simulink library "InterModuleProtocol"  (R2023b)
settings: Solver=VariableStepAuto  StartTime=0.0  StopTime=10.0  RelTol=1e-3
undefined symbols (not defined in the file or in its folder): accelerationNED, accelerationNEDXYZ, accelerationXYZ, angleOfAttack, courseOverGround, orientationQuaternion, orientationRollPitchYaw, positionLLA, positionNED, sideSlipAngle, speedOverGround, velocityNED, velocityNEDUVW, velocityPQR, velocityUVW
libraries: $bdroot x10
(part 2 of 3)

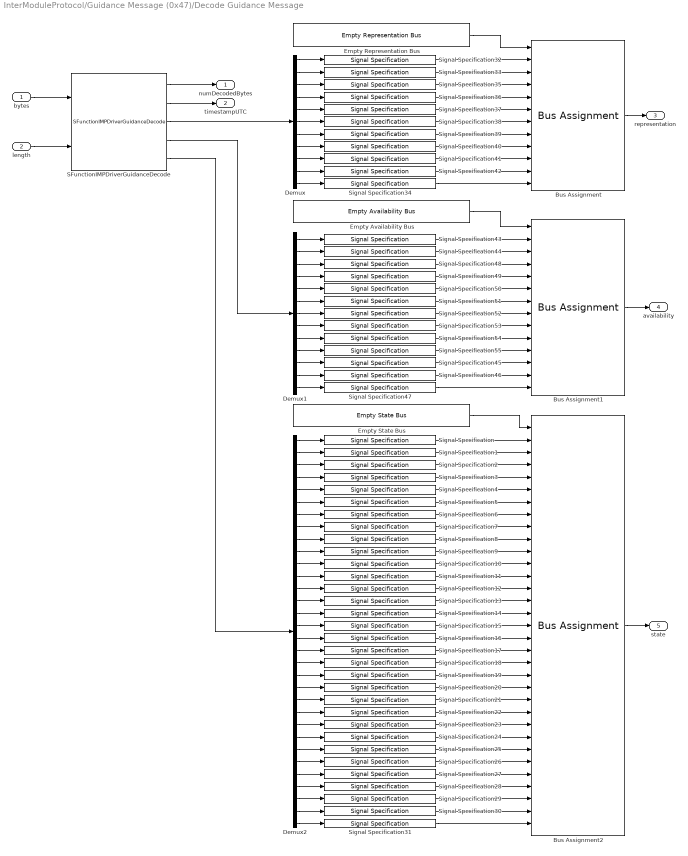
== system InterModuleProtocol/Guidance Message (0x47)/Decode Guidance Message ==
  bytes : Inport  OutDataTypeStr=uint8
  length : Inport  Port=2  OutDataTypeStr=uint32  PortDimensions=1
  Bus Assignment : BusAssignment  AssignedSignals=positionLLA,positionNED,orientationQuaternion,orientationRollPitchYaw,velocityNEDUVW,velocityPQR,accelerationNEDXYZ,courseOverGround,speedOverGround,angleOfAttack,sideSlipAngle
  Bus Assignment1 : BusAssignment  AssignedSignals=positionLLA,positionNED,orientationQuaternion,orientationRollPitchYaw,velocityNED,velocityUVW,velocityPQR,accelerationNED,accelerationXYZ,courseOverGround,speedOverGround,angleOfAttack,sideSlipAngle
  Bus Assignment2 : BusAssignment  AssignedSignals=positionLatitude,positionLongitude,positionAltitude,positionNorth,positionEast,positionDown,orientationQuaternionW,orientationQuaternionX,orientationQuaternionY,orientationQuaternionZ,orientationRoll,orientationPitch,orientationYaw,velocityNorth,velocityEast,velocityDown,velocityU,velocityV,velocityW,velocityP,velocityQ,velocityR,accelerationNorth,accelerationEast,accelerationDown,accelerationX,accelerationY,accelerationZ,courseOverGround,speedOverGround,angleOfAttack,sideSlipAngle
  Demux : Demux  Outputs=11
  Demux1 : Demux  Outputs=13
  Demux2 : Demux  Outputs=32
  Empty Availability Bus : $bdroot/Empty Availability Bus
  Empty Representation Bus : $bdroot/Empty Representation Bus
  Empty State Bus : $bdroot/Empty State Bus
  SFunctionIMPDriverGuidanceDecode : S-Function  FunctionName=SFunctionIMPDriverGuidanceDecode  Parameters=SampleTime  SFunctionDeploymentMode=off  EnableBusSupport=off  mask(Legacy Function){SFunctionSpec=void IMP_OutputDriverGuidanceDecode(uint8 u1[], uint32 u2, int32 y1[1], double y2[1], uint8 y3[11], uint8 y4[13], double y5[32]), SampleTime=-1, ShowSpec=off}
      mask prompts: SampleTime "Sample time (-1 for inherited):"; ShowSpec "Display function specification"
      mask help:
      | This block allows you to call the legacy functions specified by the following Legacy Code Tool definition:
      | def.SFunctionName = 'SFunctionIMPDriverGuidanceDecode';
      | def.OutputFcnSpec = 'void IMP_OutputDriverGuidanceDecode(uint8 u1[], uint32 u2, int32 y1[1], double y2[1], uint8 y3[11], uint8 y4[13], double y5[32])';
      | def.StartFcnSpec = 'void IMP_CreateDriverGuidanceDecode()';
      | def.TerminateFcnSpec = 'void IMP_DeleteDriverGuidanceDecode()';
      | def.HeaderFiles = {'IMP_DriverGuidanceDecode.h'};
      | def.SourceFiles = {'IMP_DriverGuidanceDecode.cpp', 'InterModuleProtocol.cpp', 'IMPConvexPolygon.cpp', 'IMPState.cpp', 'IMPStateConfiguration.cpp'};
      | def.IncPaths = {'..\..\source\InterModuleProtocol'};
      | def.SrcPaths = {'..\..\source\InterModuleProtocol'};
      | def.SampleTime = 'parameterized';
      | def.Options.useTlcWithAccel = false;
      mask Help: <p>This block was generated automatically by the Legacy Code Tool. For detailed help on this tool, call<a href="matlab:legacy_code('help')"> legacy_code('help')</a>.</p>
      mask Callback ShowSpec:
      | if strcmp(get_param(gcbh, 'ShowSpec'), 'on')
      |   set_param(gcbh, 'MaskDisplay', sprintf('fprintf(''%s'');', get_param(gcbh, 'SFunctionSpec')));
      | else
      |   set_param(gcbh, 'MaskDisplay', sprintf('fprintf(''%s'');', get_param(gcbh, 'FunctionName')));
      | end
      mask Display: fprintf('SFunctionIMPDriverGuidanceDecode');
  Signal Specification{,1,10..12,28,30..31} (8 alike) : SignalSpecification  OutDataTypeStr=double  Unit=rad  Dimensions=1
  Signal Specification{13..18,29} (7 alike) : SignalSpecification  OutDataTypeStr=double  Unit=m/s  Dimensions=1
  Signal Specification19 : SignalSpecification  OutDataTypeStr=double  Unit=rad/s  Dimensions=1
  Signal Specification{2..5} (4 alike) : SignalSpecification  OutDataTypeStr=double  Unit=m  Dimensions=1
  Signal Specification20 : SignalSpecification  OutDataTypeStr=double  Unit=rad/s  Dimensions=1
  Signal Specification21 : SignalSpecification  OutDataTypeStr=double  Unit=rad/s  Dimensions=1
  Signal Specification{22..27} (6 alike) : SignalSpecification  OutDataTypeStr=double  Unit=m/s^2  Dimensions=1
  Signal Specification{32..55} (24 alike) : SignalSpecification  OutDataTypeStr=uint8  Dimensions=1
  Signal Specification{6..9} (4 alike) : SignalSpecification  OutDataTypeStr=double  Dimensions=1
  numDecodedBytes : Outport  OutDataTypeStr=int32  PortDimensions=1  VectorParamsAs1DForOutWhenUnconnected=off
  timestampUTC : Outport  Port=2  OutDataTypeStr=double  Unit=s  PortDimensions=1  VectorParamsAs1DForOutWhenUnconnected=off
  representation : Outport  Port=3  VectorParamsAs1DForOutWhenUnconnected=off
  availability : Outport  Port=4  VectorParamsAs1DForOutWhenUnconnected=off
  state : Outport  Port=5  VectorParamsAs1DForOutWhenUnconnected=off
  wires:
  length/1 -> SFunctionIMPDriverGuidanceDecode/2
  SFunctionIMPDriverGuidanceDecode/2 -> timestampUTC/1
  bytes/1 -> SFunctionIMPDriverGuidanceDecode/1
  SFunctionIMPDriverGuidanceDecode/1 -> numDecodedBytes/1
  SFunctionIMPDriverGuidanceDecode/3 -> Demux/1
  SFunctionIMPDriverGuidanceDecode/4 -> Demux1/1
  Demux2/29 -> Signal Specification28/1
  Demux2/30 -> Signal Specification29/1
  Demux2/25 -> Signal Specification24/1
  Demux2/22 -> Signal Specification21/1
  Demux2/23 -> Signal Specification22/1
  Demux2/16 -> Signal Specification15/1
  Demux2/18 -> Signal Specification17/1
  Demux2/15 -> Signal Specification14/1
  Demux2/12 -> Signal Specification11/1
  Demux2/14 -> Signal Specification13/1
  Demux2/11 -> Signal Specification10/1
  Demux2/10 -> Signal Specification9/1
  Demux2/5 -> Signal Specification4/1
  Demux2/13 -> Signal Specification12/1
  Demux2/4 -> Signal Specification3/1
  Demux2/27 -> Signal Specification26/1
  Demux2/6 -> Signal Specification5/1
  Demux2/24 -> Signal Specification23/1
  Demux2/26 -> Signal Specification25/1
  Demux2/3 -> Signal Specification2/1
  Demux2/21 -> Signal Specification20/1
  Demux2/9 -> Signal Specification8/1
  Demux2/20 -> Signal Specification19/1
  Demux2/17 -> Signal Specification16/1
  Demux2/32 -> Signal Specification31/1
  Demux2/8 -> Signal Specification7/1
  Demux2/19 -> Signal Specification18/1
  Demux2/7 -> Signal Specification6/1
  Demux2/2 -> Signal Specification1/1
  Demux2/1 -> Signal Specification/1
  Demux2/28 -> Signal Specification27/1
  Demux2/31 -> Signal Specification30/1
  SFunctionIMPDriverGuidanceDecode/5 -> Demux2/1
  Empty Representation Bus/1 -> Bus Assignment/1
  Bus Assignment/1 -> representation/1
  Bus Assignment1/1 -> availability/1
  Empty Availability Bus/1 -> Bus Assignment1/1
  Empty State Bus/1 -> Bus Assignment2/1
  Signal Specification/1 -> Bus Assignment2/2
  Signal Specification1/1 -> Bus Assignment2/3
  Signal Specification2/1 -> Bus Assignment2/4
  Signal Specification3/1 -> Bus Assignment2/5
  Signal Specification4/1 -> Bus Assignment2/6
  Signal Specification5/1 -> Bus Assignment2/7
  Signal Specification6/1 -> Bus Assignment2/8
  Signal Specification7/1 -> Bus Assignment2/9
  Signal Specification8/1 -> Bus Assignment2/10
  Signal Specification9/1 -> Bus Assignment2/11
  Signal Specification10/1 -> Bus Assignment2/12
  Signal Specification11/1 -> Bus Assignment2/13
  Signal Specification12/1 -> Bus Assignment2/14
  Signal Specification13/1 -> Bus Assignment2/15
  Signal Specification14/1 -> Bus Assignment2/16
  Signal Specification15/1 -> Bus Assignment2/17
  Signal Specification16/1 -> Bus Assignment2/18
  Signal Specification17/1 -> Bus Assignment2/19
  Signal Specification18/1 -> Bus Assignment2/20
  Signal Specification19/1 -> Bus Assignment2/21
  Signal Specification20/1 -> Bus Assignment2/22
  Signal Specification21/1 -> Bus Assignment2/23
  Signal Specification22/1 -> Bus Assignment2/24
  Signal Specification23/1 -> Bus Assignment2/25
  Signal Specification24/1 -> Bus Assignment2/26
  Signal Specification25/1 -> Bus Assignment2/27
  Signal Specification26/1 -> Bus Assignment2/28
  Signal Specification27/1 -> Bus Assignment2/29
  Signal Specification28/1 -> Bus Assignment2/30
  Signal Specification29/1 -> Bus Assignment2/31
  Signal Specification30/1 -> Bus Assignment2/32
  Signal Specification31/1 -> Bus Assignment2/33
  Bus Assignment2/1 -> state/1
  Signal Specification32/1 -> Bus Assignment/2
  Signal Specification33/1 -> Bus Assignment/3
  Signal Specification35/1 -> Bus Assignment/4
  Signal Specification36/1 -> Bus Assignment/5
  Signal Specification37/1 -> Bus Assignment/6
  Signal Specification38/1 -> Bus Assignment/7
  Signal Specification39/1 -> Bus Assignment/8
  Signal Specification40/1 -> Bus Assignment/9
  Signal Specification41/1 -> Bus Assignment/10
  Signal Specification42/1 -> Bus Assignment/11
  Signal Specification34/1 -> Bus Assignment/12
  Demux/3 -> Signal Specification35/1
  Demux/2 -> Signal Specification33/1
  Demux/1 -> Signal Specification32/1
  Demux/4 -> Signal Specification36/1
  Demux/5 -> Signal Specification37/1
  Demux/7 -> Signal Specification39/1
  Demux/8 -> Signal Specification40/1
  Demux/9 -> Signal Specification41/1
  Demux/10 -> Signal Specification42/1
  Demux/11 -> Signal Specification34/1
  Demux/6 -> Signal Specification38/1
  Signal Specification43/1 -> Bus Assignment1/2
  Signal Specification44/1 -> Bus Assignment1/3
  Signal Specification48/1 -> Bus Assignment1/4
  Signal Specification49/1 -> Bus Assignment1/5
  Signal Specification50/1 -> Bus Assignment1/6
  Signal Specification51/1 -> Bus Assignment1/7
  Signal Specification52/1 -> Bus Assignment1/8
  Signal Specification53/1 -> Bus Assignment1/9
  Signal Specification54/1 -> Bus Assignment1/10
  Signal Specification55/1 -> Bus Assignment1/11
  Signal Specification45/1 -> Bus Assignment1/12
  Signal Specification46/1 -> Bus Assignment1/13
  Signal Specification47/1 -> Bus Assignment1/14
  Demux1/12 -> Signal Specification46/1
  Demux1/11 -> Signal Specification45/1
  Demux1/10 -> Signal Specification55/1
  Demux1/9 -> Signal Specification54/1
  Demux1/8 -> Signal Specification53/1
  Demux1/6 -> Signal Specification51/1
  Demux1/5 -> Signal Specification50/1
  Demux1/4 -> Signal Specification49/1
  Demux1/3 -> Signal Specification48/1
  Demux1/2 -> Signal Specification44/1
  Demux1/1 -> Signal Specification43/1
  Demux1/7 -> Signal Specification52/1
  Demux1/13 -> Signal Specification47/1

== system InterModuleProtocol/Guidance Message (0x47)/Encode Guidance Message ==
  timestampUTC : Inport  OutDataTypeStr=double  Unit=s  PortDimensions=1
  representation : Inport  Port=2
  availability : Inport  Port=3
  state : Inport  Port=4
  Bus Selector : BusSelector  OutputSignals=positionLLA,positionNED,orientationQuaternion,orientationRollPitchYaw,velocityNEDUVW,velocityPQR,accelerationNEDXYZ,courseOverGround,speedOverGround,angleOfAttack,sideSlipAngle  OutputAsBus=on
  Bus Selector1 : BusSelector  OutputSignals=positionLLA,positionNED,orientationQuaternion,orientationRollPitchYaw,velocityNED,velocityUVW,velocityPQR,accelerationNED,accelerationXYZ,courseOverGround,speedOverGround,angleOfAttack,sideSlipAngle  OutputAsBus=on
  Bus Selector2 : BusSelector  OutputSignals=positionLatitude,positionLongitude,positionAltitude,positionNorth,positionEast,positionDown,orientationQuaternionW,orientationQuaternionX,orientationQuaternionY,orientationQuaternionZ,orientationRoll,orientationPitch,orientationYaw,velocityNorth,velocityEast,velocityDown,velocityU,velocityV,velocityW,velocityP,velocityQ,velocityR,accelerationNorth,accelerationEast,accelerationDown,accelerationX,accelerationY,accelerationZ,courseOverGround,speedOverGround,angleOfAttack,sideSlipAngle  OutputAsBus=on
  Bus to Vector : BusToVector
  Bus to Vector1 : BusToVector
  Bus to Vector2 : BusToVector
  Data Type Conversion : DataTypeConversion  OutDataTypeStr=uint8  SaturateOnIntegerOverflow=off  RndMeth=Floor
  Data Type Conversion1 : DataTypeConversion  OutDataTypeStr=uint8  SaturateOnIntegerOverflow=off  RndMeth=Floor
  Data Type Conversion2 : DataTypeConversion  OutDataTypeStr=double  SaturateOnIntegerOverflow=off  RndMeth=Floor
  SFunctionIMPDriverGuidanceEncode : S-Function  FunctionName=SFunctionIMPDriverGuidanceEncode  Parameters=SParameter1, SampleTime  SFunctionDeploymentMode=off  EnableBusSupport=off  mask(Legacy Function){SFunctionSpec=void IMP_OutputDriverGuidanceEncode(uint8 y1[p1], uint32 y2[1], uint32 p1, double u1, uint8 u2[11], uint8 u3[13], double u4[32]), SParameter1=uint32(reshape(outputBufferSize, [1 1])), SampleTime=-1, ShowSpec=off}
      mask prompts: SParameter1 "P1:"; SampleTime "Sample time (-1 for inherited):"; ShowSpec "Display function specification"
      mask help:
      | This block allows you to call the legacy functions specified by the following Legacy Code Tool definition:
      | def.SFunctionName = 'SFunctionIMPDriverGuidanceEncode';
      | def.OutputFcnSpec = 'void IMP_OutputDriverGuidanceEncode(uint8 y1[p1], uint32 y2[1], uint32 p1, double u1, uint8 u2[11], uint8 u3[13], double u4[32])';
      | def.StartFcnSpec = 'void IMP_CreateDriverGuidanceEncode()';
      | def.TerminateFcnSpec = 'void IMP_DeleteDriverGuidanceEncode()';
      | def.HeaderFiles = {'IMP_DriverGuidanceEncode.h'};
      | def.SourceFiles = {'IMP_DriverGuidanceEncode.cpp', 'InterModuleProtocol.cpp', 'IMPConvexPolygon.cpp', 'IMPState.cpp', 'IMPStateConfiguration.cpp'};
      | def.IncPaths = {'..\..\source\InterModuleProtocol'};
      | def.SrcPaths = {'..\..\source\InterModuleProtocol'};
      | def.SampleTime = 'parameterized';
      | def.Options.useTlcWithAccel = false;
      mask Help: <p>This block was generated automatically by the Legacy Code Tool. For detailed help on this tool, call<a href="matlab:legacy_code('help')"> legacy_code('help')</a>.</p>
      mask Callback ShowSpec:
      | if strcmp(get_param(gcbh, 'ShowSpec'), 'on')
      |   set_param(gcbh, 'MaskDisplay', sprintf('fprintf(''%s'');', get_param(gcbh, 'SFunctionSpec')));
      | else
      |   set_param(gcbh, 'MaskDisplay', sprintf('fprintf(''%s'');', get_param(gcbh, 'FunctionName')));
      | end
      mask Display: fprintf('SFunctionIMPDriverGuidanceEncode');
  bytes : Outport  OutDataTypeStr=uint8  PortDimensions=outputBufferSize  VectorParamsAs1DForOutWhenUnconnected=off
  length : Outport  Port=2  OutDataTypeStr=uint32  PortDimensions=1  VectorParamsAs1DForOutWhenUnconnected=off
  wires:
  timestampUTC/1 -> SFunctionIMPDriverGuidanceEncode/1
  SFunctionIMPDriverGuidanceEncode/1 -> bytes/1
  SFunctionIMPDriverGuidanceEncode/2 -> length/1
  representation/1 -> Bus Selector/1
  Bus Selector/1 -> Bus to Vector/1
  Bus to Vector/1 -> Data Type Conversion/1
  Bus Selector1/1 -> Bus to Vector1/1
  Bus Selector2/1 -> Bus to Vector2/1
  Bus to Vector1/1 -> Data Type Conversion1/1
  Bus to Vector2/1 -> Data Type Conversion2/1
  availability/1 -> Bus Selector1/1
  state/1 -> Bus Selector2/1
  Data Type Conversion/1 -> SFunctionIMPDriverGuidanceEncode/2
  Data Type Conversion1/1 -> SFunctionIMPDriverGuidanceEncode/3
  Data Type Conversion2/1 -> SFunctionIMPDriverGuidanceEncode/4

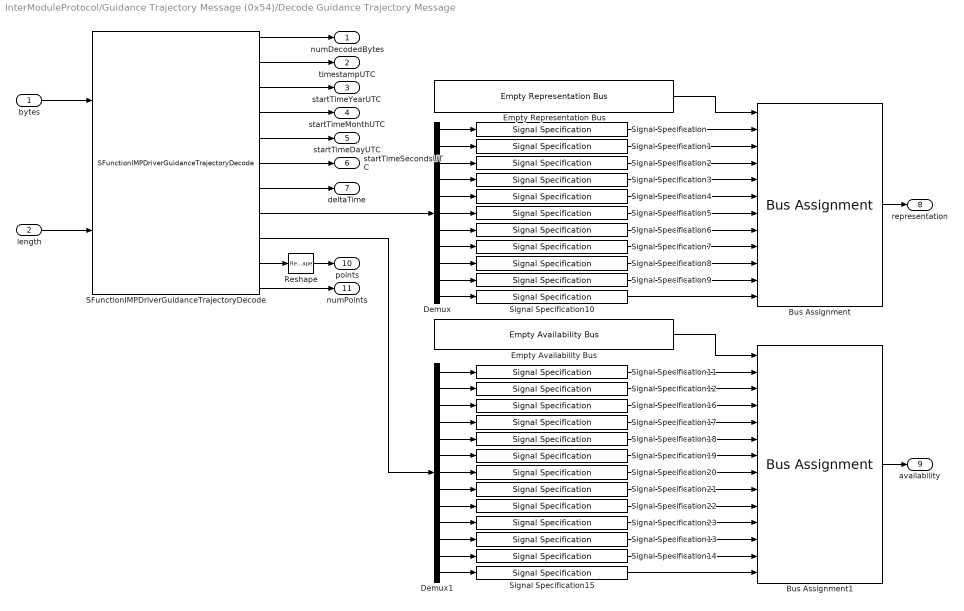
== system InterModuleProtocol/Guidance Trajectory Message (0x54)/Decode Guidance Trajectory Message ==
  bytes : Inport  OutDataTypeStr=uint8
  length : Inport  Port=2  OutDataTypeStr=uint32  PortDimensions=1
  Bus Assignment : BusAssignment  AssignedSignals=positionLLA,positionNED,orientationQuaternion,orientationRollPitchYaw,velocityNEDUVW,velocityPQR,accelerationNEDXYZ,courseOverGround,speedOverGround,angleOfAttack,sideSlipAngle
  Bus Assignment1 : BusAssignment  AssignedSignals=positionLLA,positionNED,orientationQuaternion,orientationRollPitchYaw,velocityNED,velocityUVW,velocityPQR,accelerationNED,accelerationXYZ,courseOverGround,speedOverGround,angleOfAttack,sideSlipAngle
  Demux : Demux  Outputs=11
  Demux1 : Demux  Outputs=13
  Empty Availability Bus : $bdroot/Empty Availability Bus
  Empty Representation Bus : $bdroot/Empty Representation Bus
  Reshape : Reshape  OutputDimensionality=Customize  OutputDimensions=[32,maxNumPoints]
  SFunctionIMPDriverGuidanceTrajectoryDecode : S-Function  FunctionName=SFunctionIMPDriverGuidanceTrajectoryDecode  Parameters=SParameter1, SampleTime  SFunctionDeploymentMode=off  EnableBusSupport=off  mask(Legacy Function){SFunctionSpec=void IMP_OutputDriverGuidanceTrajectoryDecode(uint8 u1[], uint32 u2, int32 y1[1], double y2[1], int32 y3[1], int32 y4[1], int32 y5[1], double y6[1], double y7[1], uint8 y8[11], uint8 y9[13], double y10[32*p1], uint32 p1, uint32 y11[1]), SParameter1=uint32(reshape(maxNumPoints, [1 1])), SampleTime=-1, ShowSpec=off}
      mask prompts: SParameter1 "P1:"; SampleTime "Sample time (-1 for inherited):"; ShowSpec "Display function specification"
      mask help:
      | This block allows you to call the legacy functions specified by the following Legacy Code Tool definition:
      | def.SFunctionName = 'SFunctionIMPDriverGuidanceTrajectoryDecode';
      | def.OutputFcnSpec = 'void IMP_OutputDriverGuidanceTrajectoryDecode(uint8 u1[], uint32 u2, int32 y1[1], double y2[1], int32 y3[1], int32 y4[1], int32 y5[1], double y6[1], double y7[1], uint8 y8[11], uint8 y9[13], double y10[32*p1], uint32 p1, uint32 y11[1])';
      | def.StartFcnSpec = 'void IMP_CreateDriverGuidanceTrajectoryDecode()';
      | def.TerminateFcnSpec = 'void IMP_DeleteDriverGuidanceTrajectoryDecode()';
      | def.HeaderFiles = {'IMP_DriverGuidanceTrajectoryDecode.h'};
      | def.SourceFiles = {'IMP_DriverGuidanceTrajectoryDecode.cpp', 'InterModuleProtocol.cpp', 'IMPConvexPolygon.cpp', 'IMPState.cpp', 'IMPStateConfiguration.cpp'};
      | def.IncPaths = {'..\..\source\InterModuleProtocol'};
      | def.SrcPaths = {'..\..\source\InterModuleProtocol'};
      | def.SampleTime = 'parameterized';
      | def.Options.useTlcWithAccel = false;
      mask Help: <p>This block was generated automatically by the Legacy Code Tool. For detailed help on this tool, call<a href="matlab:legacy_code('help')"> legacy_code('help')</a>.</p>
      mask Callback ShowSpec:
      | if strcmp(get_param(gcbh, 'ShowSpec'), 'on')
      |   set_param(gcbh, 'MaskDisplay', sprintf('fprintf(''%s'');', get_param(gcbh, 'SFunctionSpec')));
      | else
      |   set_param(gcbh, 'MaskDisplay', sprintf('fprintf(''%s'');', get_param(gcbh, 'FunctionName')));
      | end
      mask Display: fprintf('SFunctionIMPDriverGuidanceTrajectoryDecode');
  Signal Specification{,1..23} (24 alike) : SignalSpecification  OutDataTypeStr=uint8  Dimensions=1
  numDecodedBytes : Outport  OutDataTypeStr=int32  PortDimensions=1  VectorParamsAs1DForOutWhenUnconnected=off
  timestampUTC : Outport  Port=2  OutDataTypeStr=double  Unit=s  PortDimensions=1  VectorParamsAs1DForOutWhenUnconnected=off
  startTimeYearUTC : Outport  Port=3  OutDataTypeStr=int32  PortDimensions=1  VectorParamsAs1DForOutWhenUnconnected=off
  startTimeMonthUTC : Outport  Port=4  OutDataTypeStr=int32  PortDimensions=1  VectorParamsAs1DForOutWhenUnconnected=off
  startTimeDayUTC : Outport  Port=5  OutDataTypeStr=int32  PortDimensions=1  VectorParamsAs1DForOutWhenUnconnected=off
  startTimeSecondsUTC : Outport  Port=6  OutDataTypeStr=double  Unit=s  PortDimensions=1  VectorParamsAs1DForOutWhenUnconnected=off
  deltaTime : Outport  Port=7  OutDataTypeStr=double  Unit=s  PortDimensions=1  VectorParamsAs1DForOutWhenUnconnected=off
  representation : Outport  Port=8  VectorParamsAs1DForOutWhenUnconnected=off
  availability : Outport  Port=9  VectorParamsAs1DForOutWhenUnconnected=off
  points : Outport  Port=10  OutDataTypeStr=double  PortDimensions=[32, maxNumPoints]  VectorParamsAs1DForOutWhenUnconnected=off
  numPoints : Outport  Port=11  OutDataTypeStr=uint32  PortDimensions=1  VectorParamsAs1DForOutWhenUnconnected=off
  wires:
  SFunctionIMPDriverGuidanceTrajectoryDecode/5 -> startTimeDayUTC/1
  SFunctionIMPDriverGuidanceTrajectoryDecode/4 -> startTimeMonthUTC/1
  SFunctionIMPDriverGuidanceTrajectoryDecode/2 -> timestampUTC/1
  length/1 -> SFunctionIMPDriverGuidanceTrajectoryDecode/2
  bytes/1 -> SFunctionIMPDriverGuidanceTrajectoryDecode/1
  SFunctionIMPDriverGuidanceTrajectoryDecode/1 -> numDecodedBytes/1
  SFunctionIMPDriverGuidanceTrajectoryDecode/7 -> deltaTime/1
  SFunctionIMPDriverGuidanceTrajectoryDecode/3 -> startTimeYearUTC/1
  SFunctionIMPDriverGuidanceTrajectoryDecode/6 -> startTimeSecondsUTC/1
  Reshape/1 -> points/1
  SFunctionIMPDriverGuidanceTrajectoryDecode/10 -> Reshape/1
  SFunctionIMPDriverGuidanceTrajectoryDecode/11 -> numPoints/1
  Signal Specification/1 -> Bus Assignment/2
  Signal Specification5/1 -> Bus Assignment/7
  Signal Specification8/1 -> Bus Assignment/10
  Signal Specification4/1 -> Bus Assignment/6
  Signal Specification3/1 -> Bus Assignment/5
  Signal Specification6/1 -> Bus Assignment/8
  Signal Specification2/1 -> Bus Assignment/4
  Signal Specification15/1 -> Bus Assignment1/14
  Signal Specification22/1 -> Bus Assignment1/10
  Signal Specification23/1 -> Bus Assignment1/11
  Signal Specification13/1 -> Bus Assignment1/12
  Signal Specification21/1 -> Bus Assignment1/9
  Signal Specification19/1 -> Bus Assignment1/7
  Signal Specification18/1 -> Bus Assignment1/6
  Signal Specification16/1 -> Bus Assignment1/4
  Signal Specification12/1 -> Bus Assignment1/3
  Demux/3 -> Signal Specification2/1
  Demux/10 -> Signal Specification9/1
  Demux/7 -> Signal Specification6/1
  Signal Specification9/1 -> Bus Assignment/11
  Demux/4 -> Signal Specification3/1
  SFunctionIMPDriverGuidanceTrajectoryDecode/9 -> Demux1/1
  Signal Specification20/1 -> Bus Assignment1/8
  SFunctionIMPDriverGuidanceTrajectoryDecode/8 -> Demux/1
  Signal Specification11/1 -> Bus Assignment1/2
  Demux/11 -> Signal Specification10/1
  Demux/6 -> Signal Specification5/1
  Demux/8 -> Signal Specification7/1
  Demux1/6 -> Signal Specification19/1
  Demux1/7 -> Signal Specification20/1
  Demux1/4 -> Signal Specification17/1
  Demux1/2 -> Signal Specification12/1
  Signal Specification14/1 -> Bus Assignment1/13
  Demux1/13 -> Signal Specification15/1
  Demux1/11 -> Signal Specification13/1
  Signal Specification7/1 -> Bus Assignment/9
  Empty Availability Bus/1 -> Bus Assignment1/1
  Signal Specification1/1 -> Bus Assignment/3
  Demux/1 -> Signal Specification/1
  Demux1/10 -> Signal Specification23/1
  Signal Specification10/1 -> Bus Assignment/12
  Demux1/1 -> Signal Specification11/1
  Demux1/3 -> Signal Specification16/1
  Demux1/5 -> Signal Specification18/1
  Demux/9 -> Signal Specification8/1
  Demux1/8 -> Signal Specification21/1
  Bus Assignment1/1 -> availability/1
  Demux1/9 -> Signal Specification22/1
  Demux/2 -> Signal Specification1/1
  Demux1/12 -> Signal Specification14/1
  Empty Representation Bus/1 -> Bus Assignment/1
  Demux/5 -> Signal Specification4/1
  Bus Assignment/1 -> representation/1
  Signal Specification17/1 -> Bus Assignment1/5

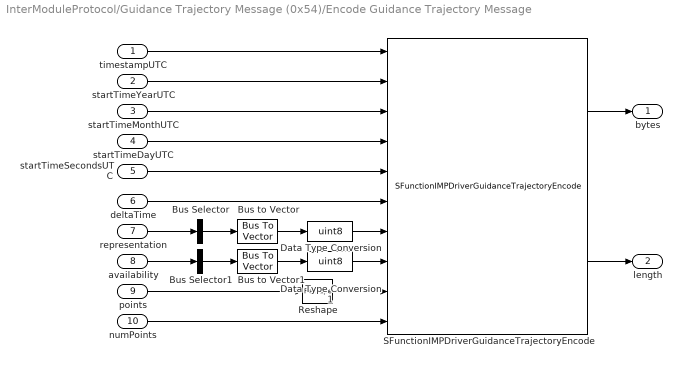
== system InterModuleProtocol/Guidance Trajectory Message (0x54)/Encode Guidance Trajectory Message ==
  timestampUTC : Inport  OutDataTypeStr=double  Unit=s  PortDimensions=1
  startTimeYearUTC : Inport  Port=2  OutDataTypeStr=int32  PortDimensions=1
  startTimeMonthUTC : Inport  Port=3  OutDataTypeStr=int32  PortDimensions=1
  startTimeDayUTC : Inport  Port=4  OutDataTypeStr=int32  PortDimensions=1
  startTimeSecondsUTC : Inport  Port=5  OutDataTypeStr=double  Unit=s  PortDimensions=1
  deltaTime : Inport  Port=6  OutDataTypeStr=double  Unit=s  PortDimensions=1
  representation : Inport  Port=7
  availability : Inport  Port=8
  points : Inport  Port=9  OutDataTypeStr=double  PortDimensions=[32, maxNumPoints]
  numPoints : Inport  Port=10  OutDataTypeStr=uint32  PortDimensions=1
  Bus Selector : BusSelector  OutputSignals=positionLLA,positionNED,orientationQuaternion,orientationRollPitchYaw,velocityNEDUVW,velocityPQR,accelerationNEDXYZ,courseOverGround,speedOverGround,angleOfAttack,sideSlipAngle  OutputAsBus=on
  Bus Selector1 : BusSelector  OutputSignals=positionLLA,positionNED,orientationQuaternion,orientationRollPitchYaw,velocityNED,velocityUVW,velocityPQR,accelerationNED,accelerationXYZ,courseOverGround,speedOverGround,angleOfAttack,sideSlipAngle  OutputAsBus=on
  Bus to Vector : BusToVector
  Bus to Vector1 : BusToVector
  Data Type Conversion : DataTypeConversion  OutDataTypeStr=uint8  SaturateOnIntegerOverflow=off  RndMeth=Floor
  Data Type Conversion1 : DataTypeConversion  OutDataTypeStr=uint8  SaturateOnIntegerOverflow=off  RndMeth=Floor
  Reshape : Reshape  OutputDimensionality=Customize  OutputDimensions=[32*maxNumPoints,1]
  SFunctionIMPDriverGuidanceTrajectoryEncode : S-Function  FunctionName=SFunctionIMPDriverGuidanceTrajectoryEncode  Parameters=SParameter1, SParameter2, SampleTime  SFunctionDeploymentMode=off  EnableBusSupport=off  mask(Legacy Function){SFunctionSpec=void IMP_OutputDriverGuidanceTrajectoryEncode(uint8 y1[p1], uint32 y2[1], uint32 p1, double u1, int32 u2, int32 u3, int32 u4, double u5, double u6, uint8 u7[11], uint8 u8[13], double u9[32*p2], uint32 p2, uint32 u10), SParameter1=uint32(reshape(outputBufferSize, [1 1])), SParameter2=uint32(reshape(maxNumPoints, [1 1])), SampleTime=-1, ShowSpec=off}
      mask prompts: SParameter1 "P1:"; SParameter2 "P2:"; SampleTime "Sample time (-1 for inherited):"; ShowSpec "Display function specification"
      mask help:
      | This block allows you to call the legacy functions specified by the following Legacy Code Tool definition:
      | def.SFunctionName = 'SFunctionIMPDriverGuidanceTrajectoryEncode';
      | def.OutputFcnSpec = 'void IMP_OutputDriverGuidanceTrajectoryEncode(uint8 y1[p1], uint32 y2[1], uint32 p1, double u1, int32 u2, int32 u3, int32 u4, double u5, double u6, uint8 u7[11], uint8 u8[13], double u9[32*p2], uint32 p2, uint32 u10)';
      | def.StartFcnSpec = 'void IMP_CreateDriverGuidanceTrajectoryEncode()';
      | def.TerminateFcnSpec = 'void IMP_DeleteDriverGuidanceTrajectoryEncode()';
      | def.HeaderFiles = {'IMP_DriverGuidanceTrajectoryEncode.h'};
      | def.SourceFiles = {'IMP_DriverGuidanceTrajectoryEncode.cpp', 'InterModuleProtocol.cpp', 'IMPConvexPolygon.cpp', 'IMPState.cpp', 'IMPStateConfiguration.cpp'};
      | def.IncPaths = {'..\..\source\InterModuleProtocol'};
      | def.SrcPaths = {'..\..\source\InterModuleProtocol'};
      | def.SampleTime = 'parameterized';
      | def.Options.useTlcWithAccel = false;
      mask Help: <p>This block was generated automatically by the Legacy Code Tool. For detailed help on this tool, call<a href="matlab:legacy_code('help')"> legacy_code('help')</a>.</p>
      mask Callback ShowSpec:
      | if strcmp(get_param(gcbh, 'ShowSpec'), 'on')
      |   set_param(gcbh, 'MaskDisplay', sprintf('fprintf(''%s'');', get_param(gcbh, 'SFunctionSpec')));
      | else
      |   set_param(gcbh, 'MaskDisplay', sprintf('fprintf(''%s'');', get_param(gcbh, 'FunctionName')));
      | end
      mask Display: fprintf('SFunctionIMPDriverGuidanceTrajectoryEncode');
  bytes : Outport  OutDataTypeStr=uint8  VectorParamsAs1DForOutWhenUnconnected=off
  length : Outport  Port=2  OutDataTypeStr=uint32  PortDimensions=1  VectorParamsAs1DForOutWhenUnconnected=off
  wires:
  SFunctionIMPDriverGuidanceTrajectoryEncode/1 -> bytes/1
  timestampUTC/1 -> SFunctionIMPDriverGuidanceTrajectoryEncode/1
  deltaTime/1 -> SFunctionIMPDriverGuidanceTrajectoryEncode/6
  SFunctionIMPDriverGuidanceTrajectoryEncode/2 -> length/1
  points/1 -> Reshape/1
  startTimeYearUTC/1 -> SFunctionIMPDriverGuidanceTrajectoryEncode/2
  startTimeMonthUTC/1 -> SFunctionIMPDriverGuidanceTrajectoryEncode/3
  startTimeDayUTC/1 -> SFunctionIMPDriverGuidanceTrajectoryEncode/4
  startTimeSecondsUTC/1 -> SFunctionIMPDriverGuidanceTrajectoryEncode/5
  Reshape/1 -> SFunctionIMPDriverGuidanceTrajectoryEncode/9
  numPoints/1 -> SFunctionIMPDriverGuidanceTrajectoryEncode/10
  representation/1 -> Bus Selector/1
  Bus Selector/1 -> Bus to Vector/1
  Bus to Vector1/1 -> Data Type Conversion1/1
  Data Type Conversion/1 -> SFunctionIMPDriverGuidanceTrajectoryEncode/7
  availability/1 -> Bus Selector1/1
  Data Type Conversion1/1 -> SFunctionIMPDriverGuidanceTrajectoryEncode/8
  Bus to Vector/1 -> Data Type Conversion/1
  Bus Selector1/1 -> Bus to Vector1/1

== system InterModuleProtocol/Info Request Message (0x00)/Decode Info Request Message ==
  bytes : Inport  OutDataTypeStr=uint8
  length : Inport  Port=2  OutDataTypeStr=uint32  PortDimensions=1
  SFunctionIMPDriverInfoRequestDecode : S-Function  FunctionName=SFunctionIMPDriverInfoRequestDecode  Parameters=SampleTime  SFunctionDeploymentMode=off  EnableBusSupport=off  mask(Legacy Function){SFunctionSpec=void IMP_OutputDriverInfoRequestDecode(uint8 u1[], uint32 u2, int32 y1[1], double y2[1]), SampleTime=-1, ShowSpec=on}
      mask prompts: SampleTime "Sample time (-1 for inherited):"; ShowSpec "Display function specification"
      mask help:
      | This block allows you to call the legacy functions specified by the following Legacy Code Tool definition:
      | def.SFunctionName = 'SFunctionIMPDriverInfoRequestDecode';
      | def.OutputFcnSpec = 'void IMP_OutputDriverInfoRequestDecode(uint8 u1[], uint32 u2, int32 y1[1], double y2[1])';
      | def.StartFcnSpec = 'void IMP_CreateDriverInfoRequestDecode()';
      | def.TerminateFcnSpec = 'void IMP_DeleteDriverInfoRequestDecode()';
      | def.HeaderFiles = {'IMP_DriverInfoRequestDecode.h'};
      | def.SourceFiles = {'IMP_DriverInfoRequestDecode.cpp', 'InterModuleProtocol.cpp', 'IMPConvexPolygon.cpp', 'IMPState.cpp', 'IMPStateConfiguration.cpp'};
      | def.IncPaths = {'..\..\source\InterModuleProtocol'};
      | def.SrcPaths = {'..\..\source\InterModuleProtocol'};
      | def.SampleTime = 'parameterized';
      | def.Options.useTlcWithAccel = false;
      mask Help: <p>This block was generated automatically by the Legacy Code Tool. For detailed help on this tool, call<a href="matlab:legacy_code('help')"> legacy_code('help')</a>.</p>
      mask Callback ShowSpec:
      | if strcmp(get_param(gcbh, 'ShowSpec'), 'on')
      |   set_param(gcbh, 'MaskDisplay', sprintf('fprintf(''%s'');', get_param(gcbh, 'SFunctionSpec')));
      | else
      |   set_param(gcbh, 'MaskDisplay', sprintf('fprintf(''%s'');', get_param(gcbh, 'FunctionName')));
      | end
      mask Display: fprintf('void IMP_OutputDriverInfoRequestDecode(uint8 u1[], uint32 u2, int32 y1[1], double y2[1])');
  numDecodedBytes : Outport  OutDataTypeStr=int32  PortDimensions=1  VectorParamsAs1DForOutWhenUnconnected=off
  timestampUTC : Outport  Port=2  OutDataTypeStr=double  Unit=s  PortDimensions=1  VectorParamsAs1DForOutWhenUnconnected=off
  wires:
  SFunctionIMPDriverInfoRequestDecode/2 -> timestampUTC/1
  bytes/1 -> SFunctionIMPDriverInfoRequestDecode/1
  length/1 -> SFunctionIMPDriverInfoRequestDecode/2
  SFunctionIMPDriverInfoRequestDecode/1 -> numDecodedBytes/1

== system InterModuleProtocol/Info Request Message (0x00)/Encode Info Request Message ==
  timestampUTC : Inport  OutDataTypeStr=double  Unit=s  PortDimensions=1
  SFunctionIMPDriverInfoRequestEncode : S-Function  FunctionName=SFunctionIMPDriverInfoRequestEncode  Parameters=SParameter1, SampleTime  SFunctionDeploymentMode=off  EnableBusSupport=off  mask(Legacy Function){SFunctionSpec=void IMP_OutputDriverInfoRequestEncode(uint8 y1[p1], uint32 y2[1], uint32 p1, double u1), SParameter1=uint32(reshape(outputBufferSize, [1 1])), SampleTime=-1, ShowSpec=on}
      mask prompts: SParameter1 "P1:"; SampleTime "Sample time (-1 for inherited):"; ShowSpec "Display function specification"
      mask help:
      | This block allows you to call the legacy functions specified by the following Legacy Code Tool definition:
      | def.SFunctionName = 'SFunctionIMPDriverInfoRequestEncode';
      | def.OutputFcnSpec = 'void IMP_OutputDriverInfoRequestEncode(uint8 y1[p1], uint32 y2[1], uint32 p1, double u1)';
      | def.StartFcnSpec = 'void IMP_CreateDriverInfoRequestEncode()';
      | def.TerminateFcnSpec = 'void IMP_DeleteDriverInfoRequestEncode()';
      | def.HeaderFiles = {'IMP_DriverInfoRequestEncode.h'};
      | def.SourceFiles = {'IMP_DriverInfoRequestEncode.cpp', 'InterModuleProtocol.cpp', 'IMPConvexPolygon.cpp', 'IMPState.cpp', 'IMPStateConfiguration.cpp'};
      | def.IncPaths = {'..\..\source\InterModuleProtocol'};
      | def.SrcPaths = {'..\..\source\InterModuleProtocol'};
      | def.SampleTime = 'parameterized';
      | def.Options.useTlcWithAccel = false;
      mask Help: <p>This block was generated automatically by the Legacy Code Tool. For detailed help on this tool, call<a href="matlab:legacy_code('help')"> legacy_code('help')</a>.</p>
      mask Callback ShowSpec:
      | if strcmp(get_param(gcbh, 'ShowSpec'), 'on')
      |   set_param(gcbh, 'MaskDisplay', sprintf('fprintf(''%s'');', get_param(gcbh, 'SFunctionSpec')));
      | else
      |   set_param(gcbh, 'MaskDisplay', sprintf('fprintf(''%s'');', get_param(gcbh, 'FunctionName')));
      | end
      mask Display: fprintf('void IMP_OutputDriverInfoRequestEncode(uint8 y1[p1], uint32 y2[1], uint32 p1, double u1)');
  bytes : Outport  OutDataTypeStr=uint8  PortDimensions=outputBufferSize  VectorParamsAs1DForOutWhenUnconnected=off
  length : Outport  Port=2  OutDataTypeStr=uint32  PortDimensions=1  VectorParamsAs1DForOutWhenUnconnected=off
  wires:
  timestampUTC/1 -> SFunctionIMPDriverInfoRequestEncode/1
  SFunctionIMPDriverInfoRequestEncode/2 -> length/1
  SFunctionIMPDriverInfoRequestEncode/1 -> bytes/1

== system InterModuleProtocol/Info Response Message (0x01)/Decode Info Response Message ==
  bytes : Inport  OutDataTypeStr=uint8
  length : Inport  Port=2  OutDataTypeStr=uint32  PortDimensions=1
  ASCII to String : ASCIIToString
  ASCII to String1 : ASCIIToString
  SFunctionIMPDriverInfoResponseDecode : S-Function  FunctionName=SFunctionIMPDriverInfoResponseDecode  Parameters=SParameter1, SampleTime  SFunctionDeploymentMode=off  EnableBusSupport=off  mask(Legacy Function){SFunctionSpec=void IMP_OutputDriverInfoResponseDecode(uint8 u1[], uint32 u2, int32 y1[1], double y2[1], double y3[3], double y4[3], uint8 y5[p1], uint8 y6[p1], uint32 p1), SParameter1=uint32(reshape(maxTextLength, [1 1])), SampleTime=-1, ShowSpec=off}
      mask prompts: SParameter1 "P1:"; SampleTime "Sample time (-1 for inherited):"; ShowSpec "Display function specification"
      mask help:
      | This block allows you to call the legacy functions specified by the following Legacy Code Tool definition:
      | def.SFunctionName = 'SFunctionIMPDriverInfoResponseDecode';
      | def.OutputFcnSpec = 'void IMP_OutputDriverInfoResponseDecode(uint8 u1[], uint32 u2, int32 y1[1], double y2[1], double y3[3], double y4[3], uint8 y5[p1], uint8 y6[p1], uint32 p1)';
      | def.StartFcnSpec = 'void IMP_CreateDriverInfoResponseDecode()';
      | def.TerminateFcnSpec = 'void IMP_DeleteDriverInfoResponseDecode()';
      | def.HeaderFiles = {'IMP_DriverInfoResponseDecode.h'};
      | def.SourceFiles = {'IMP_DriverInfoResponseDecode.cpp', 'InterModuleProtocol.cpp', 'IMPConvexPolygon.cpp', 'IMPState.cpp', 'IMPStateConfiguration.cpp'};
      | def.IncPaths = {'..\..\source\InterModuleProtocol'};
      | def.SrcPaths = {'..\..\source\InterModuleProtocol'};
      | def.SampleTime = 'parameterized';
      | def.Options.useTlcWithAccel = false;
      mask Help: <p>This block was generated automatically by the Legacy Code Tool. For detailed help on this tool, call<a href="matlab:legacy_code('help')"> legacy_code('help')</a>.</p>
      mask Callback ShowSpec:
      | if strcmp(get_param(gcbh, 'ShowSpec'), 'on')
      |   set_param(gcbh, 'MaskDisplay', sprintf('fprintf(''%s'');', get_param(gcbh, 'SFunctionSpec')));
      | else
      |   set_param(gcbh, 'MaskDisplay', sprintf('fprintf(''%s'');', get_param(gcbh, 'FunctionName')));
      | end
      mask Display: fprintf('SFunctionIMPDriverInfoResponseDecode');
  numDecodedBytes : Outport  OutDataTypeStr=int32  PortDimensions=1  VectorParamsAs1DForOutWhenUnconnected=off
  timestampUTC : Outport  Port=2  OutDataTypeStr=double  Unit=s  PortDimensions=1  VectorParamsAs1DForOutWhenUnconnected=off
  cuboidDimension : Outport  Port=3  OutDataTypeStr=double  Unit=m  PortDimensions=3  VectorParamsAs1DForOutWhenUnconnected=off
  cuboidOffset : Outport  Port=4  OutDataTypeStr=double  Unit=m  PortDimensions=3  VectorParamsAs1DForOutWhenUnconnected=off
  textVehicleName : Outport  Port=5  VectorParamsAs1DForOutWhenUnconnected=off
  textDescription : Outport  Port=6  VectorParamsAs1DForOutWhenUnconnected=off
  wires:
  SFunctionIMPDriverInfoResponseDecode/4 -> cuboidOffset/1
  length/1 -> SFunctionIMPDriverInfoResponseDecode/2
  SFunctionIMPDriverInfoResponseDecode/1 -> numDecodedBytes/1
  SFunctionIMPDriverInfoResponseDecode/6 -> ASCII to String1/1
  SFunctionIMPDriverInfoResponseDecode/5 -> ASCII to String/1
  SFunctionIMPDriverInfoResponseDecode/3 -> cuboidDimension/1
  SFunctionIMPDriverInfoResponseDecode/2 -> timestampUTC/1
  bytes/1 -> SFunctionIMPDriverInfoResponseDecode/1
  ASCII to String/1 -> textVehicleName/1
  ASCII to String1/1 -> textDescription/1

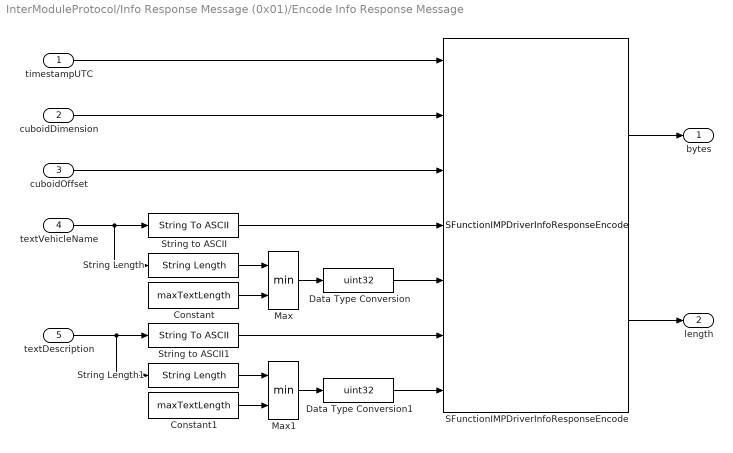
== system InterModuleProtocol/Info Response Message (0x01)/Encode Info Response Message ==
  timestampUTC : Inport  OutDataTypeStr=double  Unit=s  PortDimensions=1
  cuboidDimension : Inport  Port=2  OutDataTypeStr=double  Unit=m  PortDimensions=3
  cuboidOffset : Inport  Port=3  OutDataTypeStr=double  Unit=m  PortDimensions=3
  textVehicleName : Inport  Port=4
  textDescription : Inport  Port=5
  Constant : Constant  Value=maxTextLength
  Constant1 : Constant  Value=maxTextLength
  Data Type Conversion : DataTypeConversion  OutDataTypeStr=uint32  SaturateOnIntegerOverflow=off  RndMeth=Floor
  Data Type Conversion1 : DataTypeConversion  OutDataTypeStr=uint32  SaturateOnIntegerOverflow=off  RndMeth=Floor
  Max : MinMax  Inputs=2
  Max1 : MinMax  Inputs=2
  SFunctionIMPDriverInfoResponseEncode : S-Function  FunctionName=SFunctionIMPDriverInfoResponseEncode  Parameters=SParameter1, SParameter2, SampleTime  SFunctionDeploymentMode=off  EnableBusSupport=off  mask(Legacy Function){SFunctionSpec=void IMP_OutputDriverInfoResponseEncode(uint8 y1[p1], uint32 y2[1], uint32 p1, double u1, double u2[3], double u3[3], uint8 u4[p2], uint32 u5, uint8 u6[p2], uint32 u7, uint32 p2), SParameter1=uint32(reshape(outputBufferSize, [1 1])), SParameter2=uint32(reshape(maxTextLength, [1 1])), SampleTime=-1, ShowSpec=off}
      mask prompts: SParameter1 "P1:"; SParameter2 "P2:"; SampleTime "Sample time (-1 for inherited):"; ShowSpec "Display function specification"
      mask help:
      | This block allows you to call the legacy functions specified by the following Legacy Code Tool definition:
      | def.SFunctionName = 'SFunctionIMPDriverInfoResponseEncode';
      | def.OutputFcnSpec = 'void IMP_OutputDriverInfoResponseEncode(uint8 y1[p1], uint32 y2[1], uint32 p1, double u1, double u2[3], double u3[3], uint8 u4[p2], uint32 u5, uint8 u6[p2], uint32 u7, uint32 p2)';
      | def.StartFcnSpec = 'void IMP_CreateDriverInfoResponseEncode()';
      | def.TerminateFcnSpec = 'void IMP_DeleteDriverInfoResponseEncode()';
      | def.HeaderFiles = {'IMP_DriverInfoResponseEncode.h'};
      | def.SourceFiles = {'IMP_DriverInfoResponseEncode.cpp', 'InterModuleProtocol.cpp', 'IMPConvexPolygon.cpp', 'IMPState.cpp', 'IMPStateConfiguration.cpp'};
      | def.IncPaths = {'..\..\source\InterModuleProtocol'};
      | def.SrcPaths = {'..\..\source\InterModuleProtocol'};
      | def.SampleTime = 'parameterized';
      | def.Options.useTlcWithAccel = false;
      mask Help: <p>This block was generated automatically by the Legacy Code Tool. For detailed help on this tool, call<a href="matlab:legacy_code('help')"> legacy_code('help')</a>.</p>
      mask Callback ShowSpec:
      | if strcmp(get_param(gcbh, 'ShowSpec'), 'on')
      |   set_param(gcbh, 'MaskDisplay', sprintf('fprintf(''%s'');', get_param(gcbh, 'SFunctionSpec')));
      | else
      |   set_param(gcbh, 'MaskDisplay', sprintf('fprintf(''%s'');', get_param(gcbh, 'FunctionName')));
      | end
      mask Display: fprintf('SFunctionIMPDriverInfoResponseEncode');
  String Length : StringLength
  String Length1 : StringLength
  String to ASCII : StringToASCII  OutputVectorSize=maxTextLength
  String to ASCII1 : StringToASCII  OutputVectorSize=maxTextLength
  bytes : Outport  OutDataTypeStr=uint8  PortDimensions=outputBufferSize  VectorParamsAs1DForOutWhenUnconnected=off
  length : Outport  Port=2  OutDataTypeStr=uint32  PortDimensions=1  VectorParamsAs1DForOutWhenUnconnected=off
  wires:
  SFunctionIMPDriverInfoResponseEncode/1 -> bytes/1
  cuboidOffset/1 -> SFunctionIMPDriverInfoResponseEncode/3
  textDescription/1 -> String Length1/1, String to ASCII1/1
  cuboidDimension/1 -> SFunctionIMPDriverInfoResponseEncode/2
  timestampUTC/1 -> SFunctionIMPDriverInfoResponseEncode/1
  SFunctionIMPDriverInfoResponseEncode/2 -> length/1
  textVehicleName/1 -> String Length/1, String to ASCII/1
  String to ASCII/1 -> SFunctionIMPDriverInfoResponseEncode/4
  String to ASCII1/1 -> SFunctionIMPDriverInfoResponseEncode/6
  Max/1 -> Data Type Conversion/1
  Constant/1 -> Max/2
  String Length/1 -> Max/1
  Data Type Conversion/1 -> SFunctionIMPDriverInfoResponseEncode/5
  String Length1/1 -> Max1/1
  Constant1/1 -> Max1/2
  Max1/1 -> Data Type Conversion1/1
  Data Type Conversion1/1 -> SFunctionIMPDriverInfoResponseEncode/7

== system InterModuleProtocol/Log Message (0x4C)/Decode Log Message ==
  bytes : Inport
  length : Inport  Port=2
  ASCII to String : ASCIIToString
  SFunctionIMPDriverLogDecode : S-Function  FunctionName=SFunctionIMPDriverLogDecode  Parameters=SParameter1, SampleTime  SFunctionDeploymentMode=off  EnableBusSupport=off  mask(Legacy Function){SFunctionSpec=void IMP_OutputDriverLogDecode(uint8 u1[], uint32 u2, int32 y1[1], double y2[1], uint8 y3[3], uint8 y4[p1], uint32 p1), SParameter1=uint32(reshape(maxTextLength, [1 1])), SampleTime=-1, ShowSpec=off}
      mask prompts: SParameter1 "P1:"; SampleTime "Sample time (-1 for inherited):"; ShowSpec "Display function specification"
      mask help:
      | This block allows you to call the legacy functions specified by the following Legacy Code Tool definition:
      | def.SFunctionName = 'SFunctionIMPDriverLogDecode';
      | def.OutputFcnSpec = 'void IMP_OutputDriverLogDecode(uint8 u1[], uint32 u2, int32 y1[1], double y2[1], uint8 y3[3], uint8 y4[p1], uint32 p1)';
      | def.StartFcnSpec = 'void IMP_CreateDriverLogDecode()';
      | def.TerminateFcnSpec = 'void IMP_DeleteDriverLogDecode()';
      | def.HeaderFiles = {'IMP_DriverLogDecode.h'};
      | def.SourceFiles = {'IMP_DriverLogDecode.cpp', 'InterModuleProtocol.cpp', 'IMPConvexPolygon.cpp', 'IMPState.cpp', 'IMPStateConfiguration.cpp'};
      | def.IncPaths = {'..\..\source\InterModuleProtocol'};
      | def.SrcPaths = {'..\..\source\InterModuleProtocol'};
      | def.SampleTime = 'parameterized';
      | def.Options.useTlcWithAccel = false;
      mask Help: <p>This block was generated automatically by the Legacy Code Tool. For detailed help on this tool, call<a href="matlab:legacy_code('help')"> legacy_code('help')</a>.</p>
      mask Callback ShowSpec:
      | if strcmp(get_param(gcbh, 'ShowSpec'), 'on')
      |   set_param(gcbh, 'MaskDisplay', sprintf('fprintf(''%s'');', get_param(gcbh, 'SFunctionSpec')));
      | else
      |   set_param(gcbh, 'MaskDisplay', sprintf('fprintf(''%s'');', get_param(gcbh, 'FunctionName')));
      | end
      mask Display: fprintf('SFunctionIMPDriverLogDecode');
  numDecodedBytes : Outport  OutDataTypeStr=int32  PortDimensions=1  VectorParamsAs1DForOutWhenUnconnected=off
  timestampUTC : Outport  Port=2  OutDataTypeStr=double  Unit=s  PortDimensions=1  VectorParamsAs1DForOutWhenUnconnected=off
  color : Outport  Port=3  OutDataTypeStr=uint8  PortDimensions=3  VectorParamsAs1DForOutWhenUnconnected=off
  text : Outport  Port=4  VectorParamsAs1DForOutWhenUnconnected=off
  wires:
  SFunctionIMPDriverLogDecode/3 -> color/1
  bytes/1 -> SFunctionIMPDriverLogDecode/1
  SFunctionIMPDriverLogDecode/1 -> numDecodedBytes/1
  length/1 -> SFunctionIMPDriverLogDecode/2
  SFunctionIMPDriverLogDecode/2 -> timestampUTC/1
  SFunctionIMPDriverLogDecode/4 -> ASCII to String/1
  ASCII to String/1 -> text/1

== system InterModuleProtocol/Log Message (0x4C)/Encode Log Message ==
  timestampUTC : Inport  OutDataTypeStr=double  Unit=s  PortDimensions=1
  color : Inport  Port=2  OutDataTypeStr=uint8  PortDimensions=3
  text : Inport  Port=3
  Constant : Constant  Value=maxTextLength
  Data Type Conversion : DataTypeConversion  OutDataTypeStr=uint32  SaturateOnIntegerOverflow=off  RndMeth=Floor
  Max : MinMax  Inputs=2
  SFunctionIMPDriverLogEncode : S-Function  FunctionName=SFunctionIMPDriverLogEncode  Parameters=SParameter1, SParameter2, SampleTime  SFunctionDeploymentMode=off  EnableBusSupport=off  mask(Legacy Function){SFunctionSpec=void IMP_OutputDriverLogEncode(uint8 y1[p1], uint32 y2[1], uint32 p1, double u1, uint8 u2[3], uint8 u3[p2], uint32 p2, uint32 u4), SParameter1=uint32(reshape(outputBufferSize, [1 1])), SParameter2=uint32(reshape(maxTextLength, [1 1])), SampleTime=-1, ShowSpec=off}
      mask prompts: SParameter1 "P1:"; SParameter2 "P2:"; SampleTime "Sample time (-1 for inherited):"; ShowSpec "Display function specification"
      mask help:
      | This block allows you to call the legacy functions specified by the following Legacy Code Tool definition:
      | def.SFunctionName = 'SFunctionIMPDriverLogEncode';
      | def.OutputFcnSpec = 'void IMP_OutputDriverLogEncode(uint8 y1[p1], uint32 y2[1], uint32 p1, double u1, uint8 u2[3], uint8 u3[p2], uint32 p2, uint32 u4)';
      | def.StartFcnSpec = 'void IMP_CreateDriverLogEncode()';
      | def.TerminateFcnSpec = 'void IMP_DeleteDriverLogEncode()';
      | def.HeaderFiles = {'IMP_DriverLogEncode.h'};
      | def.SourceFiles = {'IMP_DriverLogEncode.cpp', 'InterModuleProtocol.cpp', 'IMPConvexPolygon.cpp', 'IMPState.cpp', 'IMPStateConfiguration.cpp'};
      | def.IncPaths = {'..\..\source\InterModuleProtocol'};
      | def.SrcPaths = {'..\..\source\InterModuleProtocol'};
      | def.SampleTime = 'parameterized';
      | def.Options.useTlcWithAccel = false;
      mask Help: <p>This block was generated automatically by the Legacy Code Tool. For detailed help on this tool, call<a href="matlab:legacy_code('help')"> legacy_code('help')</a>.</p>
      mask Callback ShowSpec:
      | if strcmp(get_param(gcbh, 'ShowSpec'), 'on')
      |   set_param(gcbh, 'MaskDisplay', sprintf('fprintf(''%s'');', get_param(gcbh, 'SFunctionSpec')));
      | else
      |   set_param(gcbh, 'MaskDisplay', sprintf('fprintf(''%s'');', get_param(gcbh, 'FunctionName')));
      | end
      mask Display: fprintf('SFunctionIMPDriverLogEncode');
  String Length : StringLength
  String to ASCII : StringToASCII  OutputVectorSize=maxTextLength
  bytes : Outport  OutDataTypeStr=uint8  PortDimensions=outputBufferSize  VectorParamsAs1DForOutWhenUnconnected=off
  length : Outport  Port=2  OutDataTypeStr=uint32  PortDimensions=1  VectorParamsAs1DForOutWhenUnconnected=off
  wires:
  text/1 -> String Length/1, String to ASCII/1
  SFunctionIMPDriverLogEncode/1 -> bytes/1
  SFunctionIMPDriverLogEncode/2 -> length/1
  timestampUTC/1 -> SFunctionIMPDriverLogEncode/1
  color/1 -> SFunctionIMPDriverLogEncode/2
  String to ASCII/1 -> SFunctionIMPDriverLogEncode/3
  String Length/1 -> Max/1
  Data Type Conversion/1 -> SFunctionIMPDriverLogEncode/4
  Constant/1 -> Max/2
  Max/1 -> Data Type Conversion/1
